simulink model "mech_transmission"  (Simulink 7.1)
settings: Solver=ode45  StartTime=0.0  StopTime=100  RelTol=1e-4  AbsTol=1e-4
PreLoadFcn:
  | load mech_transmission_data;
undefined symbols (not defined in the file or in its folder): converter_data, downtab, emap, Iei, Iint, mutable, Nf, r1, r2, radvec, thvec, uptab, vehicledata
libraries: mblibv1 x64
(part 2 of 2)

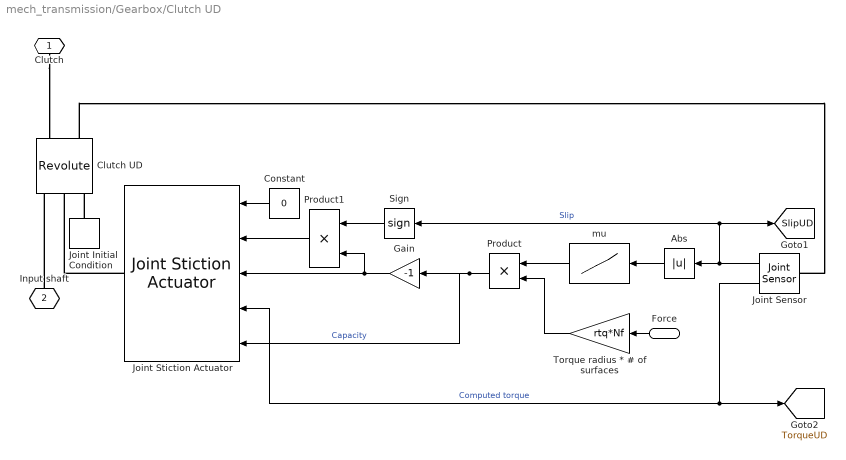
== system mech_transmission/Gearbox/Clutch UD ==
  Force : Inport  Orientation=left  OutDataType=sfix(16)  OutScaling=2^0
  Abs : Abs  Orientation=left  ZeroCross=off  SaturateOnIntegerOverflow=on
  Clutch UD : mblibv1/Joints/Revolute  Tag=Factory generic  Description=Mechanical Blockset  Orientation=up  DialogController=MECH.DynMechDlgSource  PhysicalDomain=mechanical  SubClassName=Unknown  LeftPortType=blob  RightPortType=blob  LConnTagsString=__newl0|SA1|SA2  RConnTagsString=__newr0|SA1  NumSAPorts=3  CutJoint=on  MarkAsCut=off  Primitives=revolute  PrimitiveProps=R1$WORLD$[0 0 1]$revolute  DialogClass=JointBlock  R1Axis=[0 0 1]
  Constant : Constant  Orientation=left  Value=0  OutDataType=sfix(16)  OutScaling=2^0
  Gain : Gain  Orientation=left  Gain=-1  ParameterDataType=sfix(16)  ParameterScaling=2^0  OutDataType=sfix(16)  OutScaling=2^0  SaturateOnIntegerOverflow=on  OutDataTypeStr=Inherit: Same as input  ParamDataTypeStr=Inherit: Same as input
  Joint Initial Condition : mblibv1/Sensors &  Actuators/Joint Initial Condition  Description=Mechanical Blockset  Orientation=up  DialogController=MECH.DynMechDlgSource  SystemSampleTime=-1  PhysicalDomain=Mechanical  DialogClass=InitialConditionBlock  Primitive=R1  CoordPosition=0.0  Velocity=0.0  AngleUnits=rad  ArcVelocityUnits=rad/s  CoordPositionUnits=m  VelocityUnits=m/s  InitialConditions=P1$false$0$m$rad$0$m/s$rad/s#P2$false$0$m$rad$0$m/s$rad/s#P3$false$0$m$rad$0$m/s$rad/s#R1$true$0.0$m$rad$0.0$m/s$rad/s#R2$false$0$m$rad$0$m/s$rad/s#R3$false$0$m$rad$0$m/s$rad/s#S$false$0$m$rad$0$m/s$rad/s  P1PIC=0  P1VIC=0  P2PIC=0  P2VIC=0  P3PIC=0  P3VIC=0  R1PIC=0.0  R1VIC=0.0  R2PIC=0  R2VIC=0  R3PIC=0  R3VIC=0  SPIC=0  SVIC=0
  Joint Sensor : mblibv1/Sensors &  Actuators/Joint Sensor  Description=Mechanical Blockset  Orientation=left  DialogController=MECH.DynMechDlgSource  SystemSampleTime=-1  PhysicalDomain=Mechanical  PortType=blob  Muxed=off  Pose=off  Angle=off  AngleUnits=deg  ArcVelocity=on  ArcVelocityUnits=rad/s  ArcAcceleration=off  ArcAccelerationUnits=deg/s^2  CoordPosition=on  CoordPositionUnits=m  Velocity=off  VelocityUnits=m/s  Acceleration=off  AccelerationUnits=m/s^2  Quaternion=on  QuaternionDT=off  QuaternionDDT=off  QuaternionUnits=off  OutputVector=[ 1 1 ]  ActiveIO=on  Width=2  DialogClass=MechanicalSensorBlock  Primitive=R1  Force=off  ForceUnits=N  Torque=on  TorqueUnits=N-m  ReferenceFrame=Absolute (INERTIAL)  ReactionSensedSide=Base  ReactionReferenceFrame=Absolute (World)  ReactionForce=off  ReactionForceUnits=N  ReactionMoment=off  ReactionMomentUnits=N-m
  Joint Stiction Actuator : mblibv1/Sensors &  Actuators/Joint Stiction Actuator  Description=Mechanical Blockset  Orientation=left  DialogController=MECH.DynMechDlgSource  SystemSampleTime=-1  PhysicalDomain=Mechanical  PortType=blob  ActuationStyle=Force  AngleUnits=deg  ArcVelocityUnits=deg/s  ArcAccelerationUnits=deg/s^2  CoordPositionUnits=m  VelocityUnits=m/s  AccelerationUnits=m/s^2  ForceUnits=N  TorqueUnits=N-m  ActiveIO=on  Width=5  DialogClass=EventActuatorBlock  Primitive=R1  FrictionalForceUnits=N-m  ExternalForceUnits=N-m  FrictionalTorqueUnits=N-m  ExternalTorqueUnits=N-m  LockingTolerance=1e-3
  Product : Product  Orientation=left  OutDataType=sfix(16)  OutScaling=2^0  SaturateOnIntegerOverflow=on  InputSameDT=on  OutDataTypeStr=Inherit: Same as first input
  Product1 : Product  Orientation=left  OutDataType=sfix(16)  OutScaling=2^0  SaturateOnIntegerOverflow=on  InputSameDT=on  OutDataTypeStr=Inherit: Same as first input
  Sign : Signum  Orientation=left
  Torque radius * # of surfaces : Gain  Orientation=left  Gain=rtq*Nf  ParameterDataType=sfix(16)  ParameterScaling=2^0  OutDataType=sfix(16)  OutScaling=2^0  SaturateOnIntegerOverflow=on  OutDataTypeStr=Inherit: Same as input  ParamDataTypeStr=Inherit: Same as input
  mu : Lookup  Orientation=left  InputValues=mutable(:,1)  Table=mutable(:,2)  OutDataType=sfix(16)  OutScaling=2^0  SaturateOnIntegerOverflow=on
  Clutch : PMIOPort  Orientation=down  Port=1  Side=Right
  Input shaft : PMIOPort  Orientation=up  Port=2  Side=Left
  tag scope: SlipUD=global, TorqueUD=global
  wires:
  Force/1 -> Torque radius * # of surfaces/1
  mu/1 -> Product/1
  Product1/1 -> Joint Stiction Actuator/2
  Constant/1 -> Joint Stiction Actuator/1
  Product/1 -> Gain/1, Joint Stiction Actuator/5  "Capacity"
  Torque radius * # of surfaces/1 -> Product/2
  Sign/1 -> Product1/1
  Gain/1 -> Joint Stiction Actuator/3, Product1/2
  Joint Sensor/1 -> Abs/1, Sign/1, [SlipUD]  "Slip"
  Abs/1 -> mu/1
  Joint Sensor/2 -> [TorqueUD], Joint Stiction Actuator/4  "Computed torque"
  connections:
  Input shaft/RConn1 -- Clutch UD/LConn1
  Clutch/RConn1 -- Clutch UD/RConn1
  Joint Stiction Actuator/RConn1 -- Clutch UD/LConn2
  Clutch UD/RConn2 -- Joint Sensor/LConn1
  Joint Initial Condition/RConn1 -- Clutch UD/LConn3

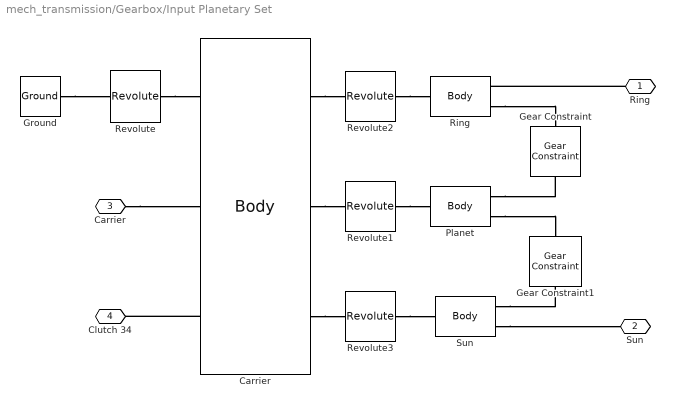
== system mech_transmission/Gearbox/Input Planetary Set ==
  Carrier : mblibv1/Bodies/Body  Tag=Factory generic  Description=Mechanical Blockset  DialogController=MECH.DynMechDlgSource  PhysicalDomain=mechanical  SubClassName=Unknown  LeftPortType=workingframe  RightPortType=workingframe  LConnTagsString=CS1|CS5|CS6  RConnTagsString=CS2|CS3|CS4  DialogClass=MechanicalBodyBlock  Mass=0.6  MassUnits=g  InertiaUnits=kg*m^2  Inertia=diag([Ic*0.07 Ic Ic])  Shape=Cylinder  ShapeDims=[1 1]  ShapeUnits=m  ShapeUse=false  Density=1  DensityUnits=kg/m^3  DensityUse=false  GraphicsMode=1  BodyColor=[0.5 0.5 0.5]  GraphicsObj=[]  AttachedToCS=1  CG=Left$CG$[-(1+R)/4 0 0]$CS3$CS3$m$[0 0 0]$Euler X-Y-Z$deg$WORLD$false  WorkingFrames=Left$CS1$[0 0 0]$WORLD$WORLD$m$[0 0 0]$Euler X-Y-Z$deg$WORLD$true#Left$CS5$[0 0 0]$CS1$CS1$m$[0 0 0]$Euler X-Y-Z$deg$WORLD$true#Left$CS6$[0 0 0]$CS1$CS1$m$[0 0 0]$Euler X-Y-Z$deg$WORLD$true#Right$CS2$[0 0 0]$CS1$CS1$m$[0 0 0]$Euler X-Y-Z$deg$WORLD$true#Right$CS3$[(1+R)/2 0 0]$CS1$CS1$m$[0 0 0]$Euler X-Y-Z$deg$WORLD$true#Right$CS4$[0 0 0]$CS1$CS1$m$[0 0 0]$Euler X-Y-Z$deg$WORLD$true  CGPos=[-(1+R)/4 0 0]  CGRot=[0 0 0]  CS0Pos=[]  CS0Rot=[]  CS1Pos=[0 0 0]  CS1Rot=[0 0 0]  CS2Pos=[0 0 0]  CS2Rot=[0 0 0]  CS3Pos=[(1+R)/2 0 0]  CS3Rot=[0 0 0]  CS4Pos=[0 0 0]  CS4Rot=[0 0 0]  CS5Pos=[0 0 0]  CS5Rot=[0 0 0]  CS6Pos=[0 0 0]  CS6Rot=[0 0 0]  CS7Pos=[]  CS7Rot=[]  CS8Pos=[]  CS8Rot=[]  CS9Pos=[]  CS9Rot=[]  CS10Pos=[]  CS10Rot=[]  CS11Pos=[]  CS11Rot=[]  CS12Pos=[]  CS12Rot=[]  CS13Pos=[]  CS13Rot=[]  CS14Pos=[]  CS14Rot=[]  CS15Pos=[]  CS15Rot=[]  CS16Pos=[]  CS16Rot=[]  CS17Pos=[]  CS17Rot=[]  CS18Pos=[]  CS18Rot=[]  CS19Pos=[]  CS19Rot=[]  CS20Pos=[]  CS20Rot=[]
  Gear Constraint : mblibv1/Constraints &  Drivers/Gear Constraint  Tag=Factory generic  Description=Mechanical Blockset  Orientation=down  DialogController=MECH.DynMechDlgSource  PhysicalDomain=mechanical  SubClassName=Unknown  LeftPortType=blob  RightPortType=blob  LConnTagsString=__newl0  RConnTagsString=__newr0  DialogClass=GearConstraint  NumSAPorts=0  BaseRadius=R  BaseRadiusUnits=m  FollowerRadius=(R-1)/2  FollowerRadiusUnits=m
  Gear Constraint1 : mblibv1/Constraints &  Drivers/Gear Constraint  Tag=Factory generic  Description=Mechanical Blockset  Orientation=up  DialogController=MECH.DynMechDlgSource  PhysicalDomain=mechanical  SubClassName=Unknown  LeftPortType=blob  RightPortType=blob  LConnTagsString=__newl0  RConnTagsString=__newr0  DialogClass=GearConstraint  NumSAPorts=0  BaseRadius=1  BaseRadiusUnits=m  FollowerRadius=(R-1)/2  FollowerRadiusUnits=m
  Ground : mblibv1/Bodies/Ground  DialogController=MECH.DynMechDlgSource  SystemSampleTime=-1  LeftPortType=env  RightPortType=workingframe  PhysicalDomain=Mechanical  DialogClass=GroundBlock  CoordPosition=[0 0 0]  CoordPositionUnits=m  StateVectorMgrId=-1  MachineId=[0 0]  ShowEnvPort=off
  Planet : mblibv1/Bodies/Body  Tag=Factory generic  Description=Mechanical Blockset  DialogController=MECH.DynMechDlgSource  PhysicalDomain=mechanical  SubClassName=Unknown  LeftPortType=workingframe  RightPortType=workingframe  LConnTagsString=CS1  RConnTagsString=CS2|CS3  DialogClass=MechanicalBodyBlock  Mass=0.01  MassUnits=g  InertiaUnits=kg*m^2  Inertia=diag([Ip*0.53 Ip*0.53 Ip])  Shape=Cylinder  ShapeDims=[1 1]  ShapeUnits=m  ShapeUse=false  Density=1  DensityUnits=kg/m^3  DensityUse=false  GraphicsMode=1  BodyColor=[0.5 0.5 0.5]  GraphicsObj=[]  AttachedToCS=1  CG=Left$CG$[0 0 0]$CS1$CS1$m$[0 0 0]$Euler X-Y-Z$deg$WORLD$false  WorkingFrames=Left$CS1$[(1+R)/2 0 0]$WORLD$WORLD$m$[0 0 0]$Euler X-Y-Z$deg$WORLD$true#Right$CS2$[0 0 0]$CS1$CS1$m$[0 0 0]$Euler X-Y-Z$deg$WORLD$true#Right$CS3$[0 0 0]$CS1$CS1$m$[0 0 0]$Euler X-Y-Z$deg$WORLD$true  CGPos=[0 0 0]  CGRot=[0 0 0]  CS0Pos=[]  CS0Rot=[]  CS1Pos=[(1+R)/2 0 0]  CS1Rot=[0 0 0]  CS2Pos=[0 0 0]  CS2Rot=[0 0 0]  CS3Pos=[0 0 0]  CS3Rot=[0 0 0]  CS4Pos=[]  CS4Rot=[]  CS5Pos=[]  CS5Rot=[]  CS6Pos=[]  CS6Rot=[]  CS7Pos=[]  CS7Rot=[]  CS8Pos=[]  CS8Rot=[]  CS9Pos=[]  CS9Rot=[]  CS10Pos=[]  CS10Rot=[]  CS11Pos=[]  CS11Rot=[]  CS12Pos=[]  CS12Rot=[]  CS13Pos=[]  CS13Rot=[]  CS14Pos=[]  CS14Rot=[]  CS15Pos=[]  CS15Rot=[]  CS16Pos=[]  CS16Rot=[]  CS17Pos=[]  CS17Rot=[]  CS18Pos=[]  CS18Rot=[]  CS19Pos=[]  CS19Rot=[]  CS20Pos=[]  CS20Rot=[]
  Revolute : mblibv1/Joints/Revolute  Tag=Factory generic  Description=Mechanical Blockset  DialogController=MECH.DynMechDlgSource  PhysicalDomain=mechanical  SubClassName=Unknown  LeftPortType=blob  RightPortType=blob  LConnTagsString=__newl0  RConnTagsString=__newr0  NumSAPorts=0  CutJoint=off  MarkAsCut=off  Primitives=revolute  PrimitiveProps=R1$WORLD$[0 0 1]$revolute  DialogClass=JointBlock  R1Axis=[0 0 1]
  Revolute1 : mblibv1/Joints/Revolute  Tag=Factory generic  Description=Mechanical Blockset  DialogController=MECH.DynMechDlgSource  PhysicalDomain=mechanical  SubClassName=Unknown  LeftPortType=blob  RightPortType=blob  LConnTagsString=__newl0  RConnTagsString=__newr0  NumSAPorts=0  CutJoint=off  MarkAsCut=off  Primitives=revolute  PrimitiveProps=R1$INERTIAL$[0 0 1]$revolute  DialogClass=JointBlock  R1Axis=[0 0 1]
  Revolute2 : mblibv1/Joints/Revolute  Tag=Factory generic  Description=Mechanical Blockset  DialogController=MECH.DynMechDlgSource  PhysicalDomain=mechanical  SubClassName=Unknown  LeftPortType=blob  RightPortType=blob  LConnTagsString=__newl0  RConnTagsString=__newr0  NumSAPorts=0  CutJoint=off  MarkAsCut=off  Primitives=revolute  PrimitiveProps=R1$INERTIAL$[0 0 1]$revolute  DialogClass=JointBlock  R1Axis=[0 0 1]
  Revolute3 : mblibv1/Joints/Revolute  Tag=Factory generic  Description=Mechanical Blockset  DialogController=MECH.DynMechDlgSource  PhysicalDomain=mechanical  SubClassName=Unknown  LeftPortType=blob  RightPortType=blob  LConnTagsString=__newl0  RConnTagsString=__newr0  NumSAPorts=0  CutJoint=off  MarkAsCut=off  Primitives=revolute  PrimitiveProps=R1$INERTIAL$[0 0 1]$revolute  DialogClass=JointBlock  R1Axis=[0 0 1]
  Ring : mblibv1/Bodies/Body  Tag=Factory generic  Description=Mechanical Blockset  DialogController=MECH.DynMechDlgSource  PhysicalDomain=mechanical  SubClassName=Unknown  LeftPortType=workingframe  RightPortType=workingframe  LConnTagsString=CS1  RConnTagsString=CS2|CS3  DialogClass=MechanicalBodyBlock  Mass=0.058  MassUnits=g  InertiaUnits=kg*m^2  Inertia=diag([0.5*Ir 0.5*Ir Ir])  Shape=Cylinder  ShapeDims=[1 1]  ShapeUnits=m  ShapeUse=false  Density=1  DensityUnits=kg/m^3  DensityUse=false  GraphicsMode=1  BodyColor=[0.5 0.5 0.5]  GraphicsObj=[]  AttachedToCS=1  CG=Left$CG$[0 0 0]$WORLD$WORLD$m$[0 0 0]$Euler X-Y-Z$deg$WORLD$false  WorkingFrames=Left$CS1$[0 0 0]$CG$CG$m$[0 0 0]$Euler X-Y-Z$deg$WORLD$true#Right$CS2$[0 0 0]$CG$CG$m$[0 0 0]$Euler X-Y-Z$deg$WORLD$true#Right$CS3$[0 0 0]$CG$CG$m$[0 0 0]$Euler X-Y-Z$deg$WORLD$true  CGPos=[0 0 0]  CGRot=[0 0 0]  CS0Pos=[]  CS0Rot=[]  CS1Pos=[0 0 0]  CS1Rot=[0 0 0]  CS2Pos=[0 0 0]  CS2Rot=[0 0 0]  CS3Pos=[0 0 0]  CS3Rot=[0 0 0]  CS4Pos=[]  CS4Rot=[]  CS5Pos=[]  CS5Rot=[]  CS6Pos=[]  CS6Rot=[]  CS7Pos=[]  CS7Rot=[]  CS8Pos=[]  CS8Rot=[]  CS9Pos=[]  CS9Rot=[]  CS10Pos=[]  CS10Rot=[]  CS11Pos=[]  CS11Rot=[]  CS12Pos=[]  CS12Rot=[]  CS13Pos=[]  CS13Rot=[]  CS14Pos=[]  CS14Rot=[]  CS15Pos=[]  CS15Rot=[]  CS16Pos=[]  CS16Rot=[]  CS17Pos=[]  CS17Rot=[]  CS18Pos=[]  CS18Rot=[]  CS19Pos=[]  CS19Rot=[]  CS20Pos=[]  CS20Rot=[]
  Sun : mblibv1/Bodies/Body  Tag=Factory generic  Description=Mechanical Blockset  DialogController=MECH.DynMechDlgSource  PhysicalDomain=mechanical  SubClassName=Unknown  LeftPortType=workingframe  RightPortType=workingframe  LConnTagsString=CS1  RConnTagsString=CS2|CS3  DialogClass=MechanicalBodyBlock  Mass=0.22  MassUnits=g  InertiaUnits=kg*m^2  Inertia=diag([Is*0.53 Is*0.53 Is])  Shape=Cylinder  ShapeDims=[1 1]  ShapeUnits=m  ShapeUse=false  Density=1  DensityUnits=kg/m^3  DensityUse=false  GraphicsMode=1  BodyColor=[0.5 0.5 0.5]  GraphicsObj=[]  AttachedToCS=1  CG=Left$CG$[0 0 0]$WORLD$WORLD$m$[0 0 0]$Euler X-Y-Z$deg$WORLD$false  WorkingFrames=Left$CS1$[0 0 0]$WORLD$WORLD$m$[0 0 0]$Euler X-Y-Z$deg$WORLD$true#Right$CS2$[0 0 0]$WORLD$WORLD$m$[0 0 0]$Euler X-Y-Z$deg$WORLD$true#Right$CS3$[0 0 0]$WORLD$WORLD$m$[0 0 0]$Euler X-Y-Z$deg$WORLD$true  CGPos=[0 0 0]  CGRot=[0 0 0]  CS0Pos=[]  CS0Rot=[]  CS1Pos=[0 0 0]  CS1Rot=[0 0 0]  CS2Pos=[0 0 0]  CS2Rot=[0 0 0]  CS3Pos=[0 0 0]  CS3Rot=[0 0 0]  CS4Pos=[]  CS4Rot=[]  CS5Pos=[]  CS5Rot=[]  CS6Pos=[]  CS6Rot=[]  CS7Pos=[]  CS7Rot=[]  CS8Pos=[]  CS8Rot=[]  CS9Pos=[]  CS9Rot=[]  CS10Pos=[]  CS10Rot=[]  CS11Pos=[]  CS11Rot=[]  CS12Pos=[]  CS12Rot=[]  CS13Pos=[]  CS13Rot=[]  CS14Pos=[]  CS14Rot=[]  CS15Pos=[]  CS15Rot=[]  CS16Pos=[]  CS16Rot=[]  CS17Pos=[]  CS17Rot=[]  CS18Pos=[]  CS18Rot=[]  CS19Pos=[]  CS19Rot=[]  CS20Pos=[]  CS20Rot=[]
  "Ring " : PMIOPort  Orientation=left  Port=1  Side=Right
  "Sun  " : PMIOPort  Orientation=left  Port=2  Side=Right
  "Carrier " : PMIOPort  Port=3  Side=Left
  Clutch 34 : PMIOPort  Port=4  Side=Right
  connections:
  Ground/RConn1 -- Revolute/LConn1
  Revolute/RConn1 -- Carrier/LConn1
  Revolute1/RConn1 -- Planet/LConn1
  Carrier/RConn2 -- Revolute1/LConn1
  Carrier/RConn1 -- Revolute2/LConn1
  Carrier/RConn3 -- Revolute3/LConn1
  Revolute2/RConn1 -- Ring/LConn1
  Revolute3/RConn1 -- Sun/LConn1
  "Ring "/RConn1 -- Ring/RConn1
  "Carrier "/RConn1 -- Carrier/LConn2
  Sun/RConn2 -- "Sun  "/RConn1
  Carrier/LConn3 -- Clutch 34/RConn1
  Ring/RConn2 -- Gear Constraint/LConn1
  Planet/RConn1 -- Gear Constraint/RConn1
  Planet/RConn2 -- Gear Constraint1/RConn1
  Sun/RConn1 -- Gear Constraint1/LConn1

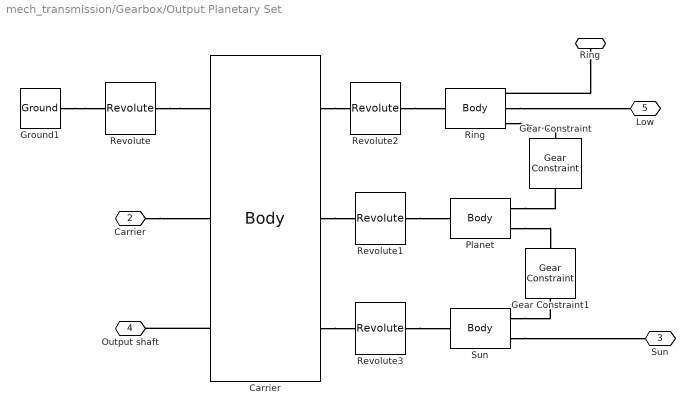
== system mech_transmission/Gearbox/Output Planetary Set ==
  Carrier : mblibv1/Bodies/Body  Tag=Factory generic  Description=Mechanical Blockset  DialogController=MECH.DynMechDlgSource  PhysicalDomain=mechanical  SubClassName=Unknown  LeftPortType=workingframe  RightPortType=workingframe  LConnTagsString=CS1|CS5|CS6  RConnTagsString=CS2|CS3|CS4  DialogClass=MechanicalBodyBlock  Mass=0.6  MassUnits=g  InertiaUnits=kg*m^2  Inertia=diag([Ic*0.07 Ic Ic])  Shape=Cylinder  ShapeDims=[1 1]  ShapeUnits=m  ShapeUse=false  Density=1  DensityUnits=kg/m^3  DensityUse=false  GraphicsMode=1  BodyColor=[0.5 0.5 0.5]  GraphicsObj=[]  AttachedToCS=1  CG=Left$CG$[0 0 1]$CS1$CS1$m$[0 0 0]$Euler X-Y-Z$deg$WORLD$false  WorkingFrames=Left$CS1$[0 0 0]$WORLD$WORLD$m$[0 0 0]$Euler X-Y-Z$deg$WORLD$true#Left$CS5$[0 0 0]$CS1$CS1$m$[0 0 0]$Euler X-Y-Z$deg$WORLD$true#Left$CS6$[0 0 0]$CS1$CS1$m$[0 0 0]$Euler X-Y-Z$deg$WORLD$true#Right$CS2$[0 0 0]$CS1$CS1$m$[0 0 0]$Euler X-Y-Z$deg$WORLD$true#Right$CS3$[(1+R)/2 0 0]$CS1$CS1$m$[0 0 0]$Euler X-Y-Z$deg$WORLD$true#Right$CS4$[0 0 0]$CS1$CS1$m$[0 0 0]$Euler X-Y-Z$deg$WORLD$true  CGPos=[0 0 1]  CGRot=[0 0 0]  CS0Pos=[]  CS0Rot=[]  CS1Pos=[0 0 0]  CS1Rot=[0 0 0]  CS2Pos=[0 0 0]  CS2Rot=[0 0 0]  CS3Pos=[(1+R)/2 0 0]  CS3Rot=[0 0 0]  CS4Pos=[0 0 0]  CS4Rot=[0 0 0]  CS5Pos=[0 0 0]  CS5Rot=[0 0 0]  CS6Pos=[0 0 0]  CS6Rot=[0 0 0]  CS7Pos=[]  CS7Rot=[]  CS8Pos=[]  CS8Rot=[]  CS9Pos=[]  CS9Rot=[]  CS10Pos=[]  CS10Rot=[]  CS11Pos=[]  CS11Rot=[]  CS12Pos=[]  CS12Rot=[]  CS13Pos=[]  CS13Rot=[]  CS14Pos=[]  CS14Rot=[]  CS15Pos=[]  CS15Rot=[]  CS16Pos=[]  CS16Rot=[]  CS17Pos=[]  CS17Rot=[]  CS18Pos=[]  CS18Rot=[]  CS19Pos=[]  CS19Rot=[]  CS20Pos=[]  CS20Rot=[]
  Gear Constraint : mblibv1/Constraints &  Drivers/Gear Constraint  Tag=Factory generic  Description=Mechanical Blockset  Orientation=down  DialogController=MECH.DynMechDlgSource  PhysicalDomain=mechanical  SubClassName=Unknown  LeftPortType=blob  RightPortType=blob  LConnTagsString=__newl0  RConnTagsString=__newr0  DialogClass=GearConstraint  NumSAPorts=0  BaseRadius=R  BaseRadiusUnits=m  FollowerRadius=(R-1)/2  FollowerRadiusUnits=m
  Gear Constraint1 : mblibv1/Constraints &  Drivers/Gear Constraint  Tag=Factory generic  Description=Mechanical Blockset  Orientation=up  DialogController=MECH.DynMechDlgSource  PhysicalDomain=mechanical  SubClassName=Unknown  LeftPortType=blob  RightPortType=blob  LConnTagsString=__newl0  RConnTagsString=__newr0  DialogClass=GearConstraint  NumSAPorts=0  BaseRadius=1  BaseRadiusUnits=m  FollowerRadius=(R-1)/2  FollowerRadiusUnits=m
  Ground1 : mblibv1/Bodies/Ground  DialogController=MECH.DynMechDlgSource  SystemSampleTime=-1  LeftPortType=env  RightPortType=workingframe  PhysicalDomain=Mechanical  DialogClass=GroundBlock  CoordPosition=[0 0 0]  CoordPositionUnits=m  StateVectorMgrId=-1  MachineId=[0 0]  ShowEnvPort=off
  Planet : mblibv1/Bodies/Body  Tag=Factory generic  Description=Mechanical Blockset  DialogController=MECH.DynMechDlgSource  PhysicalDomain=mechanical  SubClassName=Unknown  LeftPortType=workingframe  RightPortType=workingframe  LConnTagsString=CS1  RConnTagsString=CS2|CS3  DialogClass=MechanicalBodyBlock  Mass=0.01  MassUnits=g  InertiaUnits=kg*m^2  Inertia=diag([Ip*0.53 Ip*0.53 Ip])  Shape=Cylinder  ShapeDims=[1 1]  ShapeUnits=m  ShapeUse=false  Density=1  DensityUnits=kg/m^3  DensityUse=false  GraphicsMode=1  BodyColor=[0.5 0.5 0.5]  GraphicsObj=[]  AttachedToCS=1  CG=Left$CG$[0 0 1]$CS1$CS1$m$[0 0 0]$Euler X-Y-Z$deg$WORLD$false  WorkingFrames=Left$CS1$[(1+R)/2 0 0]$WORLD$WORLD$m$[0 0 0]$Euler X-Y-Z$deg$WORLD$true#Right$CS2$[0 0 0]$CS1$CS1$m$[0 0 0]$Euler X-Y-Z$deg$WORLD$true#Right$CS3$[0 0 0]$CS1$CS1$m$[0 0 0]$Euler X-Y-Z$deg$WORLD$true  CGPos=[0 0 1]  CGRot=[0 0 0]  CS0Pos=[]  CS0Rot=[]  CS1Pos=[(1+R)/2 0 0]  CS1Rot=[0 0 0]  CS2Pos=[0 0 0]  CS2Rot=[0 0 0]  CS3Pos=[0 0 0]  CS3Rot=[0 0 0]  CS4Pos=[]  CS4Rot=[]  CS5Pos=[]  CS5Rot=[]  CS6Pos=[]  CS6Rot=[]  CS7Pos=[]  CS7Rot=[]  CS8Pos=[]  CS8Rot=[]  CS9Pos=[]  CS9Rot=[]  CS10Pos=[]  CS10Rot=[]  CS11Pos=[]  CS11Rot=[]  CS12Pos=[]  CS12Rot=[]  CS13Pos=[]  CS13Rot=[]  CS14Pos=[]  CS14Rot=[]  CS15Pos=[]  CS15Rot=[]  CS16Pos=[]  CS16Rot=[]  CS17Pos=[]  CS17Rot=[]  CS18Pos=[]  CS18Rot=[]  CS19Pos=[]  CS19Rot=[]  CS20Pos=[]  CS20Rot=[]
  Revolute{,1..3} (4 alike) : mblibv1/Joints/Revolute  Tag=Factory generic  Description=Mechanical Blockset  DialogController=MECH.DynMechDlgSource  PhysicalDomain=mechanical  SubClassName=Unknown  LeftPortType=blob  RightPortType=blob  LConnTagsString=__newl0  RConnTagsString=__newr0  NumSAPorts=0  CutJoint=off  MarkAsCut=off  Primitives=revolute  PrimitiveProps=R1$WORLD$[0 0 1]$revolute  DialogClass=JointBlock  R1Axis=[0 0 1]
  Ring : mblibv1/Bodies/Body  Tag=Factory generic  Description=Mechanical Blockset  DialogController=MECH.DynMechDlgSource  PhysicalDomain=mechanical  SubClassName=Unknown  LeftPortType=workingframe  RightPortType=workingframe  LConnTagsString=CS1  RConnTagsString=CS2|CS4|CS3  DialogClass=MechanicalBodyBlock  Mass=0.08  MassUnits=g  InertiaUnits=kg*m^2  Inertia=diag([0.5*Ir 0.5*Ir Ir])  Shape=Cylinder  ShapeDims=[1 1]  ShapeUnits=m  ShapeUse=false  Density=1  DensityUnits=kg/m^3  DensityUse=false  GraphicsMode=1  BodyColor=[0.5 0.5 0.5]  GraphicsObj=[]  AttachedToCS=1  CG=Left$CG$[0 0 1]$CS1$CS1$m$[0 0 0]$Euler X-Y-Z$deg$WORLD$false  WorkingFrames=Left$CS1$[0 0 0]$WORLD$WORLD$m$[0 0 0]$Euler X-Y-Z$deg$WORLD$true#Right$CS2$[0 0 0]$CS1$CS1$m$[0 0 0]$Euler X-Y-Z$deg$WORLD$true#Right$CS4$[0 0 0]$CS1$CS1$m$[0 0 0]$Euler X-Y-Z$deg$WORLD$true#Right$CS3$[0 0 0]$CS1$CS1$m$[0 0 0]$Euler X-Y-Z$deg$WORLD$true  CGPos=[0 0 1]  CGRot=[0 0 0]  CS0Pos=[]  CS0Rot=[]  CS1Pos=[0 0 0]  CS1Rot=[0 0 0]  CS2Pos=[0 0 0]  CS2Rot=[0 0 0]  CS3Pos=[0 0 0]  CS3Rot=[0 0 0]  CS4Pos=[0 0 0]  CS4Rot=[0 0 0]  CS5Pos=[]  CS5Rot=[]  CS6Pos=[]  CS6Rot=[]  CS7Pos=[]  CS7Rot=[]  CS8Pos=[]  CS8Rot=[]  CS9Pos=[]  CS9Rot=[]  CS10Pos=[]  CS10Rot=[]  CS11Pos=[]  CS11Rot=[]  CS12Pos=[]  CS12Rot=[]  CS13Pos=[]  CS13Rot=[]  CS14Pos=[]  CS14Rot=[]  CS15Pos=[]  CS15Rot=[]  CS16Pos=[]  CS16Rot=[]  CS17Pos=[]  CS17Rot=[]  CS18Pos=[]  CS18Rot=[]  CS19Pos=[]  CS19Rot=[]  CS20Pos=[]  CS20Rot=[]
  Sun : mblibv1/Bodies/Body  Tag=Factory generic  Description=Mechanical Blockset  DialogController=MECH.DynMechDlgSource  PhysicalDomain=mechanical  SubClassName=Unknown  LeftPortType=workingframe  RightPortType=workingframe  LConnTagsString=CS1  RConnTagsString=CS2|CS3  DialogClass=MechanicalBodyBlock  Mass=0.48  MassUnits=g  InertiaUnits=kg*m^2  Inertia=diag([Is*0.53 Is*0.53 Is])  Shape=Cylinder  ShapeDims=[1 1]  ShapeUnits=m  ShapeUse=false  Density=1  DensityUnits=kg/m^3  DensityUse=false  GraphicsMode=1  BodyColor=[0.5 0.5 0.5]  GraphicsObj=[]  AttachedToCS=1  CG=Left$CG$[0 0 1]$WORLD$WORLD$m$[0 0 0]$Euler X-Y-Z$deg$WORLD$false  WorkingFrames=Left$CS1$[0 0 0]$WORLD$WORLD$m$[0 0 0]$Euler X-Y-Z$deg$WORLD$true#Right$CS2$[0 0 0]$WORLD$WORLD$m$[0 0 0]$Euler X-Y-Z$deg$WORLD$true#Right$CS3$[0 0 0]$WORLD$WORLD$m$[0 0 0]$Euler X-Y-Z$deg$WORLD$true  CGPos=[0 0 1]  CGRot=[0 0 0]  CS0Pos=[]  CS0Rot=[]  CS1Pos=[0 0 0]  CS1Rot=[0 0 0]  CS2Pos=[0 0 0]  CS2Rot=[0 0 0]  CS3Pos=[0 0 0]  CS3Rot=[0 0 0]  CS4Pos=[]  CS4Rot=[]  CS5Pos=[]  CS5Rot=[]  CS6Pos=[]  CS6Rot=[]  CS7Pos=[]  CS7Rot=[]  CS8Pos=[]  CS8Rot=[]  CS9Pos=[]  CS9Rot=[]  CS10Pos=[]  CS10Rot=[]  CS11Pos=[]  CS11Rot=[]  CS12Pos=[]  CS12Rot=[]  CS13Pos=[]  CS13Rot=[]  CS14Pos=[]  CS14Rot=[]  CS15Pos=[]  CS15Rot=[]  CS16Pos=[]  CS16Rot=[]  CS17Pos=[]  CS17Rot=[]  CS18Pos=[]  CS18Rot=[]  CS19Pos=[]  CS19Rot=[]  CS20Pos=[]  CS20Rot=[]
  "Ring " : PMIOPort  Orientation=down  Port=1  Side=Right
  "Carrier " : PMIOPort  Port=2  Side=Left
  "Sun " : PMIOPort  Orientation=left  Port=3  Side=Right
  Output shaft : PMIOPort  Port=4  Side=Left
  Low : PMIOPort  Orientation=left  Port=5  Side=Right
  connections:
  Sun/RConn2 -- "Sun "/RConn1
  "Carrier "/RConn1 -- Carrier/LConn2
  "Ring "/RConn1 -- Ring/RConn1
  Revolute3/RConn1 -- Sun/LConn1
  Revolute2/RConn1 -- Ring/LConn1
  Carrier/RConn3 -- Revolute3/LConn1
  Carrier/RConn1 -- Revolute2/LConn1
  Carrier/RConn2 -- Revolute1/LConn1
  Revolute1/RConn1 -- Planet/LConn1
  Revolute/RConn1 -- Carrier/LConn1
  Ground1/RConn1 -- Revolute/LConn1
  Ring/RConn2 -- Low/RConn1
  Carrier/LConn3 -- Output shaft/RConn1
  Ring/RConn3 -- Gear Constraint/LConn1
  Planet/RConn1 -- Gear Constraint/RConn1
  Planet/RConn2 -- Gear Constraint1/RConn1
  Sun/RConn1 -- Gear Constraint1/LConn1

== system mech_transmission/Turbine/Torbine torque ==
  Torque : Inport  OutDataType=sfix(16)  OutScaling=2^0
  Body Actuator : mblibv1/Sensors &  Actuators/Body Actuator  Description=Mechanical Blockset  Orientation=up  DialogController=MECH.DynMechDlgSource  SystemSampleTime=-1  PhysicalDomain=Mechanical  PortType=blob  ActuationStyle=Force  AngleUnits=deg  ArcVelocityUnits=deg/s  ArcAccelerationUnits=deg/s^2  CoordPositionUnits=m  VelocityUnits=m/s  AccelerationUnits=m/s^2  ForceUnits=N  TorqueUnits=N-m  ActiveIO=on  Width=3  DialogClass=MechanicalActuatorBlock  ReferenceFrame=Absolute (World)  Angle=off  CoordPosition=on  Force=off  Torque=on
  Constant : Constant  Value=0  OutDataType=sfix(16)  OutScaling=2^0
  Mux : Mux  Inputs=3
  Turbine : PMIOPort  Orientation=down  Port=1  Side=Right
  wires:
  Mux/1 -> Body Actuator/1
  Torque/1 -> Mux/3
  Constant/1 -> Mux/1, Mux/2
  connections:
  Turbine/RConn1 -- Body Actuator/RConn1

== stateflow chart  Shift_logic ==
  settings: updateMethod=DISCRETE  sampleTime=0.04
  state gear_selection/
    state gear_state [parallel]
      settings: executionOrder=1
      state fourth/
        entry: gear = 4;
      state third/
        entry: gear = 3;
      state second/
        entry: gear = 2;
      state first/
        entry: gear = 1;
      third -> fourth [order 1] : UPSHIFT34
      first -> second : UPSHIFT12
      second -> third [order 1] : UPSHIFT23
      (default) -> first
      fourth -> third : DOWNSHIFT43
      third -> second [order 2] : DOWNSHIFT32
      second -> first [order 2] : DOWNSHIFT21
    state selection_state/ [parallel]
      during: compute_thresholds;
      settings: executionOrder=2
      state downshift_confirm/
        entry: tdn = t;
      state upshift_confirm/
        entry: tup = t;
      state steady_state
      (default) -> steady_state
      steady_state -> downshift_confirm [order 2] : [vehicle_speed < down_threshold]
      steady_state -> upshift_confirm [order 1] : [vehicle_speed > up_threshold]
      downshift_confirm -> steady_state [order 1] : [vehicle_speed > down_threshold]
      (junction 13) -> steady_state
      (junction 14) -> steady_state
      upshift_confirm -> steady_state [order 2] : [vehicle_speed < up_threshold]
      upshift_confirm -> (junction 16) [order 1] : [t - tup >= Tconfirm & ...
          | vehicle_speed >= up_threshold]
      downshift_confirm -> (junction 15) [order 2] : [t - tdn >= Tconfirm & ...
          | vehicle_speed <= down_threshold]
      (junction 15) -> (junction 13) [order 1] : [gear ==4]/DOWNSHIFT43
      (junction 16) -> (junction 14) [order 3] : [gear == 3]{UPSHIFT34}
      (junction 15) -> (junction 13) [order 2] : [gear == 3]/DOWNSHIFT32
      (junction 16) -> (junction 14) [order 2] : [gear == 2]{UPSHIFT23}
      (junction 15) -> (junction 13) [order 3] : [gear == 2]/DOWNSHIFT21
      (junction 16) -> (junction 14) [order 1] : [gear == 1]{UPSHIFT12}
  data: gear output double [1..4] =1; tdn local double; tup local double; Tconfirm parameter double; down_threshold input double; up_threshold input double; vehicle_speed input double
  events: UPSHIFT12 local EITHER_EDGE_EVENT; UPSHIFT23 local EITHER_EDGE_EVENT; UPSHIFT34 local EITHER_EDGE_EVENT; DOWNSHIFT21 local EITHER_EDGE_EVENT; DOWNSHIFT32 local EITHER_EDGE_EVENT; DOWNSHIFT43 local EITHER_EDGE_EVENT; compute_thresholds output FUNCTION_CALL_EVENT
